simulink model "NDI_reference_shaping_example"  (R2023a)
settings: Solver=FixedStepAuto  StartTime=0.0  StopTime=5  FixedStep=0.001  RelTol=1e-3
settings Model: Creator=abhandari1  LastModifiedBy=abhandari1

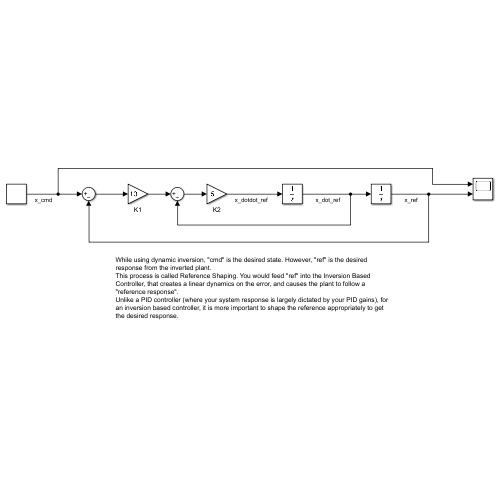
[thumbnail: Simulink's stored preview of the top-level diagram]
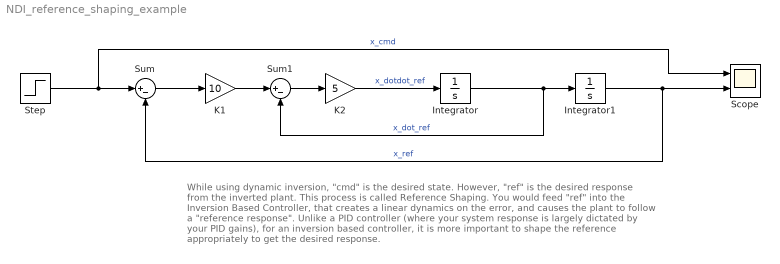
== system NDI_reference_shaping_example ==
  note: While using dynamic inversion, "cmd" is the desired state. However, "ref" is the desired response from the inverted plant.
      | This process is called Reference Shaping. You would feed "ref" into the Inversion Based Controller, that creates a linear dynamics on the error, and causes the plant to follow a "reference response".
      | Unlike a PID controller (where your system response is largely dictated by your PID gains), for an inversion based controller, it is more important to shape the reference appropriately to get the desired response.
  Integrator : Integrator
  Integrator1 : Integrator
  K1 : Gain  Gain=10
  K2 : Gain  Gain=5
  Scope : Scope  NumInputPorts=2
  Step : Step  SampleTime=0
  Sum : Sum  Inputs=|+-
  Sum1 : Sum  Inputs=|+-
  wires:
  Step/1 -> Scope/1, Sum/1  "x_cmd"
  Sum/1 -> K1/1
  K1/1 -> Sum1/1
  Sum1/1 -> K2/1
  K2/1 -> Integrator/1  "x_dotdot_ref"
  Integrator/1 -> Sum1/2, Integrator1/1  "x_dot_ref"
  Integrator1/1 -> Sum/2, Scope/2  "x_ref"
